simulink model "sim_part4"  (R2022b)
settings: Solver=VariableStepAuto  StartTime=0.0  StopTime=10.0  RelTol=1e-3
undefined symbols (not defined in the file): matA1, matB1
libraries: cstblocks x4
settings Model: Creator=alon  LastModifiedBy=binya
settings SolverCC: AlgebraicLoopSolver=TrustRegion
settings DebuggingCC: UnconnectedInputMsg=warning  UnconnectedOutputMsg=warning  UnconnectedLineMsg=warning  SFMachineParentedDataDiag=warning
settings ModelReferenceCC: EnableRefExpFcnMdlSchedulingChecks=on

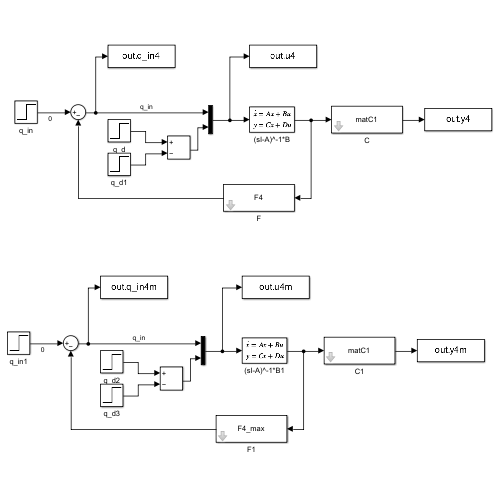
[thumbnail: Simulink's stored preview of the top-level diagram]
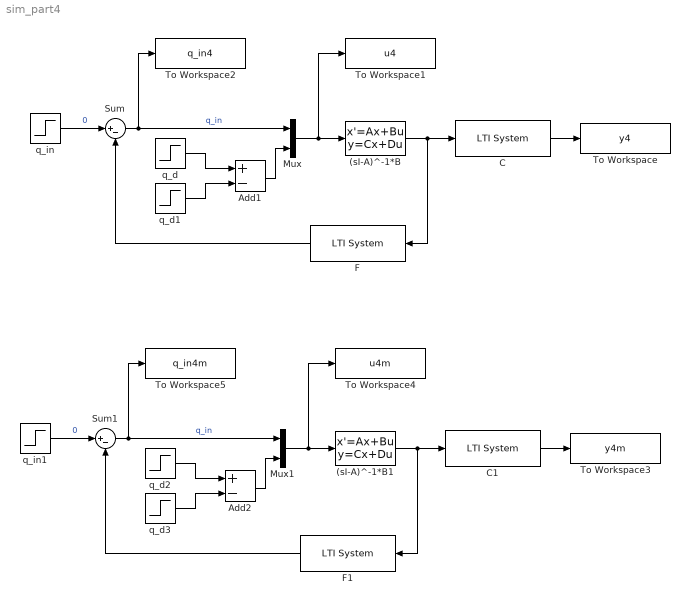
== system sim_part4 ==
  (sI-A)^-1*B : StateSpace  A=matA1  B=matB1  C=eye(3)  D=[[0 0];[0 0];[0 0]]  InitialCondition=0
  (sI-A)^-1*B1 : StateSpace  A=matA1  B=matB1  C=eye(3)  D=[[0 0];[0 0];[0 0]]  InitialCondition=0
  Add1 : Sum  Inputs=+-
  Add2 : Sum  Inputs=+-
  C : cstblocks/LTI System  sys=matC1  IC=[]
  C1 : cstblocks/LTI System  sys=matC1  IC=[]
  F : cstblocks/LTI System  sys=F4  IC=[]
  F1 : cstblocks/LTI System  sys=F4_max  IC=[]
  Mux : Mux  Inputs=2
  Mux1 : Mux  Inputs=2
  Sum : Sum  Inputs=|+-
  Sum1 : Sum  Inputs=|+-
  To Workspace : ToWorkspace  VariableName=y4  SaveFormat=Timeseries  SampleTime=-1
  To Workspace1 : ToWorkspace  VariableName=u4  SaveFormat=Timeseries  SampleTime=-1
  To Workspace2 : ToWorkspace  VariableName=q_in4  SaveFormat=Timeseries  SampleTime=-1
  To Workspace3 : ToWorkspace  VariableName=y4m  SaveFormat=Timeseries  SampleTime=-1
  To Workspace4 : ToWorkspace  VariableName=u4m  SaveFormat=Timeseries  SampleTime=-1
  To Workspace5 : ToWorkspace  VariableName=q_in4m  SaveFormat=Timeseries  SampleTime=-1
  q_d : Step  Time=0  After=12  SampleTime=0
  q_d1 : Step  Time=2.3  After=12  SampleTime=0
  q_d2 : Step  Time=0  After=12  SampleTime=0
  q_d3 : Step  Time=2.3  After=12  SampleTime=0
  q_in : Step  Time=0  After=0  SampleTime=0
  q_in1 : Step  Time=0  After=0  SampleTime=0
  wires:
  q_in/1 -> Sum/1  "0"
  q_d/1 -> Add1/1
  Add1/1 -> Mux/2
  C/1 -> To Workspace/1
  q_d1/1 -> Add1/2
  (sI-A)^-1*B/1 -> F/1, C/1
  Mux/1 -> To Workspace1/1, (sI-A)^-1*B/1
  Sum/1 -> Mux/1, To Workspace2/1  "q_in"
  F/1 -> Sum/2
  q_in1/1 -> Sum1/1  "0"
  F1/1 -> Sum1/2
  (sI-A)^-1*B1/1 -> F1/1, C1/1
  Mux1/1 -> To Workspace4/1, (sI-A)^-1*B1/1
  q_d3/1 -> Add2/2
  Sum1/1 -> Mux1/1, To Workspace5/1  "q_in"
  q_d2/1 -> Add2/1
  Add2/1 -> Mux1/2
  C1/1 -> To Workspace3/1
